simulink model "c00004M_harness"  (R2018a)
settings: Solver=FixedStepAuto  StartTime=0.0  StopTime=300  FixedStep=0.1  RelTol=1e-3
undefined symbols (not defined in the file): A1, hmax, R1, R2, sigbuilder_block, TempThreshold
(part 2 of 14)

== system c00004M_harness/Eval201 ==
  In3 : Inport
  Constant1 : Constant
  Constant2 : Constant
  Data Type Conversion2 : DataTypeConversion
  Memory3 : Memory  InitialCondition=1
  MinMax : MinMax  Inputs=3
  MinMax3 : MinMax  Inputs=2
  ROOut3 : RelationalOperator  Operator===  OutDataTypeStr=boolean  RndMeth=Simplest
  Out1 : Outport
  wires:
  Data Type Conversion2/1 -> MinMax3/1
  Memory3/1 -> MinMax3/2
  ROOut3/1 -> Data Type Conversion2/1
  MinMax3/1 -> Memory3/1, MinMax/3
  In3/1 -> ROOut3/1
  [out3] -> ROOut3/2
  MinMax/1 -> Out1/1
  Constant1/1 -> MinMax/1
  Constant2/1 -> MinMax/2

== system c00004M_harness/Eval202 ==
  In3 : Inport
  Constant1 : Constant
  Constant2 : Constant
  Data Type Conversion2 : DataTypeConversion
  Memory3 : Memory  InitialCondition=1
  MinMax : MinMax  Inputs=3
  MinMax3 : MinMax  Inputs=2
  ROOut3 : RelationalOperator  Operator===  OutDataTypeStr=boolean  RndMeth=Simplest
  Out1 : Outport
  wires:
  Data Type Conversion2/1 -> MinMax3/1
  Memory3/1 -> MinMax3/2
  ROOut3/1 -> Data Type Conversion2/1
  MinMax3/1 -> Memory3/1, MinMax/3
  In3/1 -> ROOut3/1
  [out3] -> ROOut3/2
  MinMax/1 -> Out1/1
  Constant1/1 -> MinMax/1
  Constant2/1 -> MinMax/2

== system c00004M_harness/Eval203 ==
  In3 : Inport
  Constant1 : Constant
  Constant2 : Constant
  Data Type Conversion2 : DataTypeConversion
  Memory3 : Memory  InitialCondition=1
  MinMax : MinMax  Inputs=3
  MinMax3 : MinMax  Inputs=2
  ROOut3 : RelationalOperator  Operator===  OutDataTypeStr=boolean  RndMeth=Simplest
  Out1 : Outport
  wires:
  Data Type Conversion2/1 -> MinMax3/1
  Memory3/1 -> MinMax3/2
  ROOut3/1 -> Data Type Conversion2/1
  MinMax3/1 -> Memory3/1, MinMax/3
  In3/1 -> ROOut3/1
  [out3] -> ROOut3/2
  MinMax/1 -> Out1/1
  Constant1/1 -> MinMax/1
  Constant2/1 -> MinMax/2

== system c00004M_harness/Eval204 ==
  In3 : Inport
  Constant1 : Constant
  Constant2 : Constant
  Data Type Conversion2 : DataTypeConversion
  Memory3 : Memory  InitialCondition=1
  MinMax : MinMax  Inputs=3
  MinMax3 : MinMax  Inputs=2
  ROOut3 : RelationalOperator  Operator===  OutDataTypeStr=boolean  RndMeth=Simplest
  Out1 : Outport
  wires:
  Data Type Conversion2/1 -> MinMax3/1
  Memory3/1 -> MinMax3/2
  ROOut3/1 -> Data Type Conversion2/1
  MinMax3/1 -> Memory3/1, MinMax/3
  In3/1 -> ROOut3/1
  [out3] -> ROOut3/2
  MinMax/1 -> Out1/1
  Constant1/1 -> MinMax/1
  Constant2/1 -> MinMax/2

== system c00004M_harness/Eval205 ==
  In3 : Inport
  Constant1 : Constant
  Constant2 : Constant
  Data Type Conversion2 : DataTypeConversion
  Memory3 : Memory  InitialCondition=1
  MinMax : MinMax  Inputs=3
  MinMax3 : MinMax  Inputs=2
  ROOut3 : RelationalOperator  Operator===  OutDataTypeStr=boolean  RndMeth=Simplest
  Out1 : Outport
  wires:
  Data Type Conversion2/1 -> MinMax3/1
  Memory3/1 -> MinMax3/2
  ROOut3/1 -> Data Type Conversion2/1
  MinMax3/1 -> Memory3/1, MinMax/3
  In3/1 -> ROOut3/1
  [out3] -> ROOut3/2
  MinMax/1 -> Out1/1
  Constant1/1 -> MinMax/1
  Constant2/1 -> MinMax/2

== system c00004M_harness/Eval206 ==
  In3 : Inport
  Constant1 : Constant
  Constant2 : Constant
  Data Type Conversion2 : DataTypeConversion
  Memory3 : Memory  InitialCondition=1
  MinMax : MinMax  Inputs=3
  MinMax3 : MinMax  Inputs=2
  ROOut3 : RelationalOperator  Operator===  OutDataTypeStr=boolean  RndMeth=Simplest
  Out1 : Outport
  wires:
  Data Type Conversion2/1 -> MinMax3/1
  Memory3/1 -> MinMax3/2
  ROOut3/1 -> Data Type Conversion2/1
  MinMax3/1 -> Memory3/1, MinMax/3
  In3/1 -> ROOut3/1
  [out3] -> ROOut3/2
  MinMax/1 -> Out1/1
  Constant1/1 -> MinMax/1
  Constant2/1 -> MinMax/2

== system c00004M_harness/Eval207 ==
  In3 : Inport
  Constant1 : Constant
  Constant2 : Constant
  Data Type Conversion2 : DataTypeConversion
  Memory3 : Memory  InitialCondition=1
  MinMax : MinMax  Inputs=3
  MinMax3 : MinMax  Inputs=2
  ROOut3 : RelationalOperator  Operator===  OutDataTypeStr=boolean  RndMeth=Simplest
  Out1 : Outport
  wires:
  Data Type Conversion2/1 -> MinMax3/1
  Memory3/1 -> MinMax3/2
  ROOut3/1 -> Data Type Conversion2/1
  MinMax3/1 -> Memory3/1, MinMax/3
  In3/1 -> ROOut3/1
  [out3] -> ROOut3/2
  MinMax/1 -> Out1/1
  Constant1/1 -> MinMax/1
  Constant2/1 -> MinMax/2

== system c00004M_harness/Eval208 ==
  In3 : Inport
  Constant1 : Constant
  Constant2 : Constant
  Data Type Conversion2 : DataTypeConversion
  Memory3 : Memory  InitialCondition=1
  MinMax : MinMax  Inputs=3
  MinMax3 : MinMax  Inputs=2
  ROOut3 : RelationalOperator  Operator===  OutDataTypeStr=boolean  RndMeth=Simplest
  Out1 : Outport
  wires:
  Data Type Conversion2/1 -> MinMax3/1
  Memory3/1 -> MinMax3/2
  ROOut3/1 -> Data Type Conversion2/1
  MinMax3/1 -> Memory3/1, MinMax/3
  In3/1 -> ROOut3/1
  [out3] -> ROOut3/2
  MinMax/1 -> Out1/1
  Constant1/1 -> MinMax/1
  Constant2/1 -> MinMax/2

== system c00004M_harness/Eval209 ==
  In3 : Inport
  Constant1 : Constant
  Constant2 : Constant
  Data Type Conversion2 : DataTypeConversion
  Memory3 : Memory  InitialCondition=1
  MinMax : MinMax  Inputs=3
  MinMax3 : MinMax  Inputs=2
  ROOut3 : RelationalOperator  Operator===  OutDataTypeStr=boolean  RndMeth=Simplest
  Out1 : Outport
  wires:
  Data Type Conversion2/1 -> MinMax3/1
  Memory3/1 -> MinMax3/2
  ROOut3/1 -> Data Type Conversion2/1
  MinMax3/1 -> Memory3/1, MinMax/3
  In3/1 -> ROOut3/1
  [out3] -> ROOut3/2
  MinMax/1 -> Out1/1
  Constant1/1 -> MinMax/1
  Constant2/1 -> MinMax/2

== system c00004M_harness/Eval210 ==
  In3 : Inport
  Constant1 : Constant
  Constant2 : Constant
  Data Type Conversion2 : DataTypeConversion
  Memory3 : Memory  InitialCondition=1
  MinMax : MinMax  Inputs=3
  MinMax3 : MinMax  Inputs=2
  ROOut3 : RelationalOperator  Operator===  OutDataTypeStr=boolean  RndMeth=Simplest
  Out1 : Outport
  wires:
  Data Type Conversion2/1 -> MinMax3/1
  Memory3/1 -> MinMax3/2
  ROOut3/1 -> Data Type Conversion2/1
  MinMax3/1 -> Memory3/1, MinMax/3
  In3/1 -> ROOut3/1
  [out3] -> ROOut3/2
  MinMax/1 -> Out1/1
  Constant1/1 -> MinMax/1
  Constant2/1 -> MinMax/2

== system c00004M_harness/Eval211 ==
  In3 : Inport
  Constant1 : Constant
  Constant2 : Constant
  Data Type Conversion2 : DataTypeConversion
  Memory3 : Memory  InitialCondition=1
  MinMax : MinMax  Inputs=3
  MinMax3 : MinMax  Inputs=2
  ROOut3 : RelationalOperator  Operator===  OutDataTypeStr=boolean  RndMeth=Simplest
  Out1 : Outport
  wires:
  Data Type Conversion2/1 -> MinMax3/1
  Memory3/1 -> MinMax3/2
  ROOut3/1 -> Data Type Conversion2/1
  MinMax3/1 -> Memory3/1, MinMax/3
  In3/1 -> ROOut3/1
  [out3] -> ROOut3/2
  MinMax/1 -> Out1/1
  Constant1/1 -> MinMax/1
  Constant2/1 -> MinMax/2

== system c00004M_harness/Eval212 ==
  In3 : Inport
  Constant1 : Constant
  Constant2 : Constant
  Data Type Conversion2 : DataTypeConversion
  Memory3 : Memory  InitialCondition=1
  MinMax : MinMax  Inputs=3
  MinMax3 : MinMax  Inputs=2
  ROOut3 : RelationalOperator  Operator===  OutDataTypeStr=boolean  RndMeth=Simplest
  Out1 : Outport
  wires:
  Data Type Conversion2/1 -> MinMax3/1
  Memory3/1 -> MinMax3/2
  ROOut3/1 -> Data Type Conversion2/1
  MinMax3/1 -> Memory3/1, MinMax/3
  In3/1 -> ROOut3/1
  [out3] -> ROOut3/2
  MinMax/1 -> Out1/1
  Constant1/1 -> MinMax/1
  Constant2/1 -> MinMax/2

== system c00004M_harness/Eval213 ==
  In3 : Inport
  Constant1 : Constant
  Constant2 : Constant
  Data Type Conversion2 : DataTypeConversion
  Memory3 : Memory  InitialCondition=1
  MinMax : MinMax  Inputs=3
  MinMax3 : MinMax  Inputs=2
  ROOut3 : RelationalOperator  Operator===  OutDataTypeStr=boolean  RndMeth=Simplest
  Out1 : Outport
  wires:
  Data Type Conversion2/1 -> MinMax3/1
  Memory3/1 -> MinMax3/2
  ROOut3/1 -> Data Type Conversion2/1
  MinMax3/1 -> Memory3/1, MinMax/3
  In3/1 -> ROOut3/1
  [out3] -> ROOut3/2
  MinMax/1 -> Out1/1
  Constant1/1 -> MinMax/1
  Constant2/1 -> MinMax/2

== system c00004M_harness/Eval214 ==
  In3 : Inport
  Constant1 : Constant
  Constant2 : Constant
  Data Type Conversion2 : DataTypeConversion
  Memory3 : Memory  InitialCondition=1
  MinMax : MinMax  Inputs=3
  MinMax3 : MinMax  Inputs=2
  ROOut3 : RelationalOperator  Operator===  OutDataTypeStr=boolean  RndMeth=Simplest
  Out1 : Outport
  wires:
  Data Type Conversion2/1 -> MinMax3/1
  Memory3/1 -> MinMax3/2
  ROOut3/1 -> Data Type Conversion2/1
  MinMax3/1 -> Memory3/1, MinMax/3
  In3/1 -> ROOut3/1
  [out3] -> ROOut3/2
  MinMax/1 -> Out1/1
  Constant1/1 -> MinMax/1
  Constant2/1 -> MinMax/2

== system c00004M_harness/Eval215 ==
  In3 : Inport
  Constant1 : Constant
  Constant2 : Constant
  Data Type Conversion2 : DataTypeConversion
  Memory3 : Memory  InitialCondition=1
  MinMax : MinMax  Inputs=3
  MinMax3 : MinMax  Inputs=2
  ROOut3 : RelationalOperator  Operator===  OutDataTypeStr=boolean  RndMeth=Simplest
  Out1 : Outport
  wires:
  Data Type Conversion2/1 -> MinMax3/1
  Memory3/1 -> MinMax3/2
  ROOut3/1 -> Data Type Conversion2/1
  MinMax3/1 -> Memory3/1, MinMax/3
  In3/1 -> ROOut3/1
  [out3] -> ROOut3/2
  MinMax/1 -> Out1/1
  Constant1/1 -> MinMax/1
  Constant2/1 -> MinMax/2

== system c00004M_harness/Eval216 ==
  In3 : Inport
  Constant1 : Constant
  Constant2 : Constant
  Data Type Conversion2 : DataTypeConversion
  Memory3 : Memory  InitialCondition=1
  MinMax : MinMax  Inputs=3
  MinMax3 : MinMax  Inputs=2
  ROOut3 : RelationalOperator  Operator===  OutDataTypeStr=boolean  RndMeth=Simplest
  Out1 : Outport
  wires:
  Data Type Conversion2/1 -> MinMax3/1
  Memory3/1 -> MinMax3/2
  ROOut3/1 -> Data Type Conversion2/1
  MinMax3/1 -> Memory3/1, MinMax/3
  In3/1 -> ROOut3/1
  [out3] -> ROOut3/2
  MinMax/1 -> Out1/1
  Constant1/1 -> MinMax/1
  Constant2/1 -> MinMax/2

== system c00004M_harness/Eval217 ==
  In3 : Inport
  Constant1 : Constant
  Constant2 : Constant
  Data Type Conversion2 : DataTypeConversion
  Memory3 : Memory  InitialCondition=1
  MinMax : MinMax  Inputs=3
  MinMax3 : MinMax  Inputs=2
  ROOut3 : RelationalOperator  Operator===  OutDataTypeStr=boolean  RndMeth=Simplest
  Out1 : Outport
  wires:
  Data Type Conversion2/1 -> MinMax3/1
  Memory3/1 -> MinMax3/2
  ROOut3/1 -> Data Type Conversion2/1
  MinMax3/1 -> Memory3/1, MinMax/3
  In3/1 -> ROOut3/1
  [out3] -> ROOut3/2
  MinMax/1 -> Out1/1
  Constant1/1 -> MinMax/1
  Constant2/1 -> MinMax/2

== system c00004M_harness/Eval218 ==
  In3 : Inport
  Constant1 : Constant
  Constant2 : Constant
  Data Type Conversion2 : DataTypeConversion
  Memory3 : Memory  InitialCondition=1
  MinMax : MinMax  Inputs=3
  MinMax3 : MinMax  Inputs=2
  ROOut3 : RelationalOperator  Operator===  OutDataTypeStr=boolean  RndMeth=Simplest
  Out1 : Outport
  wires:
  Data Type Conversion2/1 -> MinMax3/1
  Memory3/1 -> MinMax3/2
  ROOut3/1 -> Data Type Conversion2/1
  MinMax3/1 -> Memory3/1, MinMax/3
  In3/1 -> ROOut3/1
  [out3] -> ROOut3/2
  MinMax/1 -> Out1/1
  Constant1/1 -> MinMax/1
  Constant2/1 -> MinMax/2

== system c00004M_harness/Eval219 ==
  In3 : Inport
  Constant1 : Constant
  Constant2 : Constant
  Data Type Conversion2 : DataTypeConversion
  Memory3 : Memory  InitialCondition=1
  MinMax : MinMax  Inputs=3
  MinMax3 : MinMax  Inputs=2
  ROOut3 : RelationalOperator  Operator===  OutDataTypeStr=boolean  RndMeth=Simplest
  Out1 : Outport
  wires:
  Data Type Conversion2/1 -> MinMax3/1
  Memory3/1 -> MinMax3/2
  ROOut3/1 -> Data Type Conversion2/1
  MinMax3/1 -> Memory3/1, MinMax/3
  In3/1 -> ROOut3/1
  [out3] -> ROOut3/2
  MinMax/1 -> Out1/1
  Constant1/1 -> MinMax/1
  Constant2/1 -> MinMax/2

== system c00004M_harness/Eval220 ==
  In3 : Inport
  Constant1 : Constant
  Constant2 : Constant
  Data Type Conversion2 : DataTypeConversion
  Memory3 : Memory  InitialCondition=1
  MinMax : MinMax  Inputs=3
  MinMax3 : MinMax  Inputs=2
  ROOut3 : RelationalOperator  Operator===  OutDataTypeStr=boolean  RndMeth=Simplest
  Out1 : Outport
  wires:
  Data Type Conversion2/1 -> MinMax3/1
  Memory3/1 -> MinMax3/2
  ROOut3/1 -> Data Type Conversion2/1
  MinMax3/1 -> Memory3/1, MinMax/3
  In3/1 -> ROOut3/1
  [out3] -> ROOut3/2
  MinMax/1 -> Out1/1
  Constant1/1 -> MinMax/1
  Constant2/1 -> MinMax/2

== system c00004M_harness/Eval221 ==
  In3 : Inport
  Constant1 : Constant
  Constant2 : Constant
  Data Type Conversion2 : DataTypeConversion
  Memory3 : Memory  InitialCondition=1
  MinMax : MinMax  Inputs=3
  MinMax3 : MinMax  Inputs=2
  ROOut3 : RelationalOperator  Operator===  OutDataTypeStr=boolean  RndMeth=Simplest
  Out1 : Outport
  wires:
  Data Type Conversion2/1 -> MinMax3/1
  Memory3/1 -> MinMax3/2
  ROOut3/1 -> Data Type Conversion2/1
  MinMax3/1 -> Memory3/1, MinMax/3
  In3/1 -> ROOut3/1
  [out3] -> ROOut3/2
  MinMax/1 -> Out1/1
  Constant1/1 -> MinMax/1
  Constant2/1 -> MinMax/2

== system c00004M_harness/Eval222 ==
  In3 : Inport
  Constant1 : Constant
  Constant2 : Constant
  Data Type Conversion2 : DataTypeConversion
  Memory3 : Memory  InitialCondition=1
  MinMax : MinMax  Inputs=3
  MinMax3 : MinMax  Inputs=2
  ROOut3 : RelationalOperator  Operator===  OutDataTypeStr=boolean  RndMeth=Simplest
  Out1 : Outport
  wires:
  Data Type Conversion2/1 -> MinMax3/1
  Memory3/1 -> MinMax3/2
  ROOut3/1 -> Data Type Conversion2/1
  MinMax3/1 -> Memory3/1, MinMax/3
  In3/1 -> ROOut3/1
  [out3] -> ROOut3/2
  MinMax/1 -> Out1/1
  Constant1/1 -> MinMax/1
  Constant2/1 -> MinMax/2

== system c00004M_harness/Eval223 ==
  In3 : Inport
  Constant1 : Constant
  Constant2 : Constant
  Data Type Conversion2 : DataTypeConversion
  Memory3 : Memory  InitialCondition=1
  MinMax : MinMax  Inputs=3
  MinMax3 : MinMax  Inputs=2
  ROOut3 : RelationalOperator  Operator===  OutDataTypeStr=boolean  RndMeth=Simplest
  Out1 : Outport
  wires:
  Data Type Conversion2/1 -> MinMax3/1
  Memory3/1 -> MinMax3/2
  ROOut3/1 -> Data Type Conversion2/1
  MinMax3/1 -> Memory3/1, MinMax/3
  In3/1 -> ROOut3/1
  [out3] -> ROOut3/2
  MinMax/1 -> Out1/1
  Constant1/1 -> MinMax/1
  Constant2/1 -> MinMax/2

== system c00004M_harness/Eval224 ==
  In3 : Inport
  Constant1 : Constant
  Constant2 : Constant
  Data Type Conversion2 : DataTypeConversion
  Memory3 : Memory  InitialCondition=1
  MinMax : MinMax  Inputs=3
  MinMax3 : MinMax  Inputs=2
  ROOut3 : RelationalOperator  Operator===  OutDataTypeStr=boolean  RndMeth=Simplest
  Out1 : Outport
  wires:
  Data Type Conversion2/1 -> MinMax3/1
  Memory3/1 -> MinMax3/2
  ROOut3/1 -> Data Type Conversion2/1
  MinMax3/1 -> Memory3/1, MinMax/3
  In3/1 -> ROOut3/1
  [out3] -> ROOut3/2
  MinMax/1 -> Out1/1
  Constant1/1 -> MinMax/1
  Constant2/1 -> MinMax/2

== system c00004M_harness/Eval232 ==
  In3 : Inport
  Constant1 : Constant
  Constant2 : Constant
  Data Type Conversion2 : DataTypeConversion
  Memory3 : Memory  InitialCondition=1
  MinMax : MinMax  Inputs=3
  MinMax3 : MinMax  Inputs=2
  ROOut3 : RelationalOperator  Operator===  OutDataTypeStr=boolean  RndMeth=Simplest
  Out1 : Outport
  wires:
  Data Type Conversion2/1 -> MinMax3/1
  Memory3/1 -> MinMax3/2
  ROOut3/1 -> Data Type Conversion2/1
  MinMax3/1 -> Memory3/1, MinMax/3
  In3/1 -> ROOut3/1
  [out3] -> ROOut3/2
  MinMax/1 -> Out1/1
  Constant1/1 -> MinMax/1
  Constant2/1 -> MinMax/2

== system c00004M_harness/Eval233 ==
  In3 : Inport
  Constant1 : Constant
  Constant2 : Constant
  Data Type Conversion2 : DataTypeConversion
  Memory3 : Memory  InitialCondition=1
  MinMax : MinMax  Inputs=3
  MinMax3 : MinMax  Inputs=2
  ROOut3 : RelationalOperator  Operator===  OutDataTypeStr=boolean  RndMeth=Simplest
  Out1 : Outport
  wires:
  Data Type Conversion2/1 -> MinMax3/1
  Memory3/1 -> MinMax3/2
  ROOut3/1 -> Data Type Conversion2/1
  MinMax3/1 -> Memory3/1, MinMax/3
  In3/1 -> ROOut3/1
  [out3] -> ROOut3/2
  MinMax/1 -> Out1/1
  Constant1/1 -> MinMax/1
  Constant2/1 -> MinMax/2

== system c00004M_harness/Eval234 ==
  In3 : Inport
  Constant1 : Constant
  Constant2 : Constant
  Data Type Conversion2 : DataTypeConversion
  Memory3 : Memory  InitialCondition=1
  MinMax : MinMax  Inputs=3
  MinMax3 : MinMax  Inputs=2
  ROOut3 : RelationalOperator  Operator===  OutDataTypeStr=boolean  RndMeth=Simplest
  Out1 : Outport
  wires:
  Data Type Conversion2/1 -> MinMax3/1
  Memory3/1 -> MinMax3/2
  ROOut3/1 -> Data Type Conversion2/1
  MinMax3/1 -> Memory3/1, MinMax/3
  In3/1 -> ROOut3/1
  [out3] -> ROOut3/2
  MinMax/1 -> Out1/1
  Constant1/1 -> MinMax/1
  Constant2/1 -> MinMax/2

== system c00004M_harness/Eval235 ==
  In3 : Inport
  Constant1 : Constant
  Constant2 : Constant
  Data Type Conversion2 : DataTypeConversion
  Memory3 : Memory  InitialCondition=1
  MinMax : MinMax  Inputs=3
  MinMax3 : MinMax  Inputs=2
  ROOut3 : RelationalOperator  Operator===  OutDataTypeStr=boolean  RndMeth=Simplest
  Out1 : Outport
  wires:
  Data Type Conversion2/1 -> MinMax3/1
  Memory3/1 -> MinMax3/2
  ROOut3/1 -> Data Type Conversion2/1
  MinMax3/1 -> Memory3/1, MinMax/3
  In3/1 -> ROOut3/1
  [out3] -> ROOut3/2
  MinMax/1 -> Out1/1
  Constant1/1 -> MinMax/1
  Constant2/1 -> MinMax/2

== system c00004M_harness/Eval236 ==
  In3 : Inport
  Constant1 : Constant
  Constant2 : Constant
  Data Type Conversion2 : DataTypeConversion
  Memory3 : Memory  InitialCondition=1
  MinMax : MinMax  Inputs=3
  MinMax3 : MinMax  Inputs=2
  ROOut3 : RelationalOperator  Operator===  OutDataTypeStr=boolean  RndMeth=Simplest
  Out1 : Outport
  wires:
  Data Type Conversion2/1 -> MinMax3/1
  Memory3/1 -> MinMax3/2
  ROOut3/1 -> Data Type Conversion2/1
  MinMax3/1 -> Memory3/1, MinMax/3
  In3/1 -> ROOut3/1
  [out3] -> ROOut3/2
  MinMax/1 -> Out1/1
  Constant1/1 -> MinMax/1
  Constant2/1 -> MinMax/2

== system c00004M_harness/Eval237 ==
  In3 : Inport
  Constant1 : Constant
  Constant2 : Constant
  Data Type Conversion2 : DataTypeConversion
  Memory3 : Memory  InitialCondition=1
  MinMax : MinMax  Inputs=3
  MinMax3 : MinMax  Inputs=2
  ROOut3 : RelationalOperator  Operator===  OutDataTypeStr=boolean  RndMeth=Simplest
  Out1 : Outport
  wires:
  Data Type Conversion2/1 -> MinMax3/1
  Memory3/1 -> MinMax3/2
  ROOut3/1 -> Data Type Conversion2/1
  MinMax3/1 -> Memory3/1, MinMax/3
  In3/1 -> ROOut3/1
  [out3] -> ROOut3/2
  MinMax/1 -> Out1/1
  Constant1/1 -> MinMax/1
  Constant2/1 -> MinMax/2

== system c00004M_harness/Eval238 ==
  In3 : Inport
  Constant1 : Constant
  Constant2 : Constant
  Data Type Conversion2 : DataTypeConversion
  Memory3 : Memory  InitialCondition=1
  MinMax : MinMax  Inputs=3
  MinMax3 : MinMax  Inputs=2
  ROOut3 : RelationalOperator  Operator===  OutDataTypeStr=boolean  RndMeth=Simplest
  Out1 : Outport
  wires:
  Data Type Conversion2/1 -> MinMax3/1
  Memory3/1 -> MinMax3/2
  ROOut3/1 -> Data Type Conversion2/1
  MinMax3/1 -> Memory3/1, MinMax/3
  In3/1 -> ROOut3/1
  [out3] -> ROOut3/2
  MinMax/1 -> Out1/1
  Constant1/1 -> MinMax/1
  Constant2/1 -> MinMax/2

== system c00004M_harness/Eval239 ==
  In3 : Inport
  Constant1 : Constant
  Constant2 : Constant
  Data Type Conversion2 : DataTypeConversion
  Memory3 : Memory  InitialCondition=1
  MinMax : MinMax  Inputs=3
  MinMax3 : MinMax  Inputs=2
  ROOut3 : RelationalOperator  Operator===  OutDataTypeStr=boolean  RndMeth=Simplest
  Out1 : Outport
  wires:
  Data Type Conversion2/1 -> MinMax3/1
  Memory3/1 -> MinMax3/2
  ROOut3/1 -> Data Type Conversion2/1
  MinMax3/1 -> Memory3/1, MinMax/3
  In3/1 -> ROOut3/1
  [out3] -> ROOut3/2
  MinMax/1 -> Out1/1
  Constant1/1 -> MinMax/1
  Constant2/1 -> MinMax/2

== system c00004M_harness/Eval240 ==
  In3 : Inport
  Constant1 : Constant
  Constant2 : Constant
  Data Type Conversion2 : DataTypeConversion
  Memory3 : Memory  InitialCondition=1
  MinMax : MinMax  Inputs=3
  MinMax3 : MinMax  Inputs=2
  ROOut3 : RelationalOperator  Operator===  OutDataTypeStr=boolean  RndMeth=Simplest
  Out1 : Outport
  wires:
  Data Type Conversion2/1 -> MinMax3/1
  Memory3/1 -> MinMax3/2
  ROOut3/1 -> Data Type Conversion2/1
  MinMax3/1 -> Memory3/1, MinMax/3
  In3/1 -> ROOut3/1
  [out3] -> ROOut3/2
  MinMax/1 -> Out1/1
  Constant1/1 -> MinMax/1
  Constant2/1 -> MinMax/2

== system c00004M_harness/Eval241 ==
  In3 : Inport
  Constant1 : Constant
  Constant2 : Constant
  Data Type Conversion2 : DataTypeConversion
  Memory3 : Memory  InitialCondition=1
  MinMax : MinMax  Inputs=3
  MinMax3 : MinMax  Inputs=2
  ROOut3 : RelationalOperator  Operator===  OutDataTypeStr=boolean  RndMeth=Simplest
  Out1 : Outport
  wires:
  Data Type Conversion2/1 -> MinMax3/1
  Memory3/1 -> MinMax3/2
  ROOut3/1 -> Data Type Conversion2/1
  MinMax3/1 -> Memory3/1, MinMax/3
  In3/1 -> ROOut3/1
  [out3] -> ROOut3/2
  MinMax/1 -> Out1/1
  Constant1/1 -> MinMax/1
  Constant2/1 -> MinMax/2

== system c00004M_harness/Eval242 ==
  In3 : Inport
  Constant1 : Constant
  Constant2 : Constant
  Data Type Conversion2 : DataTypeConversion
  Memory3 : Memory  InitialCondition=1
  MinMax : MinMax  Inputs=3
  MinMax3 : MinMax  Inputs=2
  ROOut3 : RelationalOperator  Operator===  OutDataTypeStr=boolean  RndMeth=Simplest
  Out1 : Outport
  wires:
  Data Type Conversion2/1 -> MinMax3/1
  Memory3/1 -> MinMax3/2
  ROOut3/1 -> Data Type Conversion2/1
  MinMax3/1 -> Memory3/1, MinMax/3
  In3/1 -> ROOut3/1
  [out3] -> ROOut3/2
  MinMax/1 -> Out1/1
  Constant1/1 -> MinMax/1
  Constant2/1 -> MinMax/2

== system c00004M_harness/Eval243 ==
  In3 : Inport
  Constant1 : Constant
  Constant2 : Constant
  Data Type Conversion2 : DataTypeConversion
  Memory3 : Memory  InitialCondition=1
  MinMax : MinMax  Inputs=3
  MinMax3 : MinMax  Inputs=2
  ROOut3 : RelationalOperator  Operator===  OutDataTypeStr=boolean  RndMeth=Simplest
  Out1 : Outport
  wires:
  Data Type Conversion2/1 -> MinMax3/1
  Memory3/1 -> MinMax3/2
  ROOut3/1 -> Data Type Conversion2/1
  MinMax3/1 -> Memory3/1, MinMax/3
  In3/1 -> ROOut3/1
  [out3] -> ROOut3/2
  MinMax/1 -> Out1/1
  Constant1/1 -> MinMax/1
  Constant2/1 -> MinMax/2

== system c00004M_harness/Eval244 ==
  In3 : Inport
  Constant1 : Constant
  Constant2 : Constant
  Data Type Conversion2 : DataTypeConversion
  Memory3 : Memory  InitialCondition=1
  MinMax : MinMax  Inputs=3
  MinMax3 : MinMax  Inputs=2
  ROOut3 : RelationalOperator  Operator===  OutDataTypeStr=boolean  RndMeth=Simplest
  Out1 : Outport
  wires:
  Data Type Conversion2/1 -> MinMax3/1
  Memory3/1 -> MinMax3/2
  ROOut3/1 -> Data Type Conversion2/1
  MinMax3/1 -> Memory3/1, MinMax/3
  In3/1 -> ROOut3/1
  [out3] -> ROOut3/2
  MinMax/1 -> Out1/1
  Constant1/1 -> MinMax/1
  Constant2/1 -> MinMax/2

== system c00004M_harness/Eval245 ==
  In3 : Inport
  Constant1 : Constant
  Constant2 : Constant
  Data Type Conversion2 : DataTypeConversion
  Memory3 : Memory  InitialCondition=1
  MinMax : MinMax  Inputs=3
  MinMax3 : MinMax  Inputs=2
  ROOut3 : RelationalOperator  Operator===  OutDataTypeStr=boolean  RndMeth=Simplest
  Out1 : Outport
  wires:
  Data Type Conversion2/1 -> MinMax3/1
  Memory3/1 -> MinMax3/2
  ROOut3/1 -> Data Type Conversion2/1
  MinMax3/1 -> Memory3/1, MinMax/3
  In3/1 -> ROOut3/1
  [out3] -> ROOut3/2
  MinMax/1 -> Out1/1
  Constant1/1 -> MinMax/1
  Constant2/1 -> MinMax/2

== system c00004M_harness/Inputs ==
  Demux : Demux  Tag=STV Demux  Outputs=6
  FromWs : FromWorkspace  Tag=STV FromWs  VariableName=tuvar  SampleTime=0
  CT3 : Outport  Tag=STV Outport
  F3 : Outport  Tag=STV Outport  Port=2
  E3 : Outport  Tag=STV Outport  Port=3
  MR3 : Outport  Tag=STV Outport  Port=4
  T3 : Outport  Tag=STV Outport  Port=5
  EB3 : Outport  Tag=STV Outport  Port=6
  wires:
  Demux/6 -> EB3/1
  Demux/5 -> T3/1
  Demux/4 -> MR3/1
  Demux/3 -> E3/1
  Demux/2 -> F3/1
  Demux/1 -> CT3/1
  FromWs/1 -> Demux/1

== system c00004M_harness/M165 ==
  note: VALUES
      | ---------------------------------
      | ControlType = 1 | 2 | 3
      | FillTank = 0 | 1
      | EmptyTank = 0 | 1
      | ManualReference between 0 and 1
      | Tempreature between 0 and 100
      | EmergencyButton = 0 | 1
      | LiquidLevel between 0 and 1 (hmax)
  note: Inputs For Tank2
  note: NAMES
      | --------------------------------------------
      | CT1 = ControlType Tank 1
      | F1 = Fill Tank 1
      | E1 = Empty Tank 1
      | MR1 = Manual Reference Tank1
      | T1 = Temperature Tank 1
      | EB1 = Emergency Button Tank 1
      | LL1 = Liquid Level 1
  note: Inputs For Tank3
  note: Inputs For Tank1
  CT3 : Inport
  F3 : Inport  Port=2
  E3 : Inport  Port=3
  MR3 : Inport  Port=4
  T3 : Inport  Port=5
  EB3 : Inport  Port=6
  Tank3 : Subsystem
  LL3 : Outport
  wires:
  Tank3/1(LL3) -> LL3/1
  MR3/1 -> Tank3/4(MR3)
  E3/1 -> Tank3/3(E3)
  CT3/1 -> Tank3/1(CT3)
  F3/1 -> Tank3/2(F3)
  EB3/1 -> Tank3/6(EB3)
  T3/1 -> Tank3/5(T3)

== system c00004M_harness/M166 ==
  note: VALUES
      | ---------------------------------
      | ControlType = 1 | 2 | 3
      | FillTank = 0 | 1
      | EmptyTank = 0 | 1
      | ManualReference between 0 and 1
      | Tempreature between 0 and 100
      | EmergencyButton = 0 | 1
      | LiquidLevel between 0 and 1 (hmax)
  note: Inputs For Tank2
  note: NAMES
      | --------------------------------------------
      | CT1 = ControlType Tank 1
      | F1 = Fill Tank 1
      | E1 = Empty Tank 1
      | MR1 = Manual Reference Tank1
      | T1 = Temperature Tank 1
      | EB1 = Emergency Button Tank 1
      | LL1 = Liquid Level 1
  note: Inputs For Tank3
  note: Inputs For Tank1
  CT3 : Inport
  F3 : Inport  Port=2
  E3 : Inport  Port=3
  MR3 : Inport  Port=4
  T3 : Inport  Port=5
  EB3 : Inport  Port=6
  Tank3 : Subsystem
  LL3 : Outport
  wires:
  Tank3/1(LL3) -> LL3/1
  MR3/1 -> Tank3/4(MR3)
  E3/1 -> Tank3/3(E3)
  CT3/1 -> Tank3/1(CT3)
  F3/1 -> Tank3/2(F3)
  EB3/1 -> Tank3/6(EB3)
  T3/1 -> Tank3/5(T3)

== system c00004M_harness/M167 ==
  note: VALUES
      | ---------------------------------
      | ControlType = 1 | 2 | 3
      | FillTank = 0 | 1
      | EmptyTank = 0 | 1
      | ManualReference between 0 and 1
      | Tempreature between 0 and 100
      | EmergencyButton = 0 | 1
      | LiquidLevel between 0 and 1 (hmax)
  note: Inputs For Tank2
  note: NAMES
      | --------------------------------------------
      | CT1 = ControlType Tank 1
      | F1 = Fill Tank 1
      | E1 = Empty Tank 1
      | MR1 = Manual Reference Tank1
      | T1 = Temperature Tank 1
      | EB1 = Emergency Button Tank 1
      | LL1 = Liquid Level 1
  note: Inputs For Tank3
  note: Inputs For Tank1
  CT3 : Inport
  F3 : Inport  Port=2
  E3 : Inport  Port=3
  MR3 : Inport  Port=4
  T3 : Inport  Port=5
  EB3 : Inport  Port=6
  Tank3 : Subsystem
  LL3 : Outport
  wires:
  Tank3/1(LL3) -> LL3/1
  MR3/1 -> Tank3/4(MR3)
  E3/1 -> Tank3/3(E3)
  CT3/1 -> Tank3/1(CT3)
  F3/1 -> Tank3/2(F3)
  EB3/1 -> Tank3/6(EB3)
  T3/1 -> Tank3/5(T3)

== system c00004M_harness/M168 ==
  note: VALUES
      | ---------------------------------
      | ControlType = 1 | 2 | 3
      | FillTank = 0 | 1
      | EmptyTank = 0 | 1
      | ManualReference between 0 and 1
      | Tempreature between 0 and 100
      | EmergencyButton = 0 | 1
      | LiquidLevel between 0 and 1 (hmax)
  note: Inputs For Tank2
  note: NAMES
      | --------------------------------------------
      | CT1 = ControlType Tank 1
      | F1 = Fill Tank 1
      | E1 = Empty Tank 1
      | MR1 = Manual Reference Tank1
      | T1 = Temperature Tank 1
      | EB1 = Emergency Button Tank 1
      | LL1 = Liquid Level 1
  note: Inputs For Tank3
  note: Inputs For Tank1
  CT3 : Inport
  F3 : Inport  Port=2
  E3 : Inport  Port=3
  MR3 : Inport  Port=4
  T3 : Inport  Port=5
  EB3 : Inport  Port=6
  Tank3 : Subsystem
  LL3 : Outport
  wires:
  Tank3/1(LL3) -> LL3/1
  MR3/1 -> Tank3/4(MR3)
  E3/1 -> Tank3/3(E3)
  CT3/1 -> Tank3/1(CT3)
  F3/1 -> Tank3/2(F3)
  EB3/1 -> Tank3/6(EB3)
  T3/1 -> Tank3/5(T3)

== system c00004M_harness/M169 ==
  note: VALUES
      | ---------------------------------
      | ControlType = 1 | 2 | 3
      | FillTank = 0 | 1
      | EmptyTank = 0 | 1
      | ManualReference between 0 and 1
      | Tempreature between 0 and 100
      | EmergencyButton = 0 | 1
      | LiquidLevel between 0 and 1 (hmax)
  note: Inputs For Tank2
  note: NAMES
      | --------------------------------------------
      | CT1 = ControlType Tank 1
      | F1 = Fill Tank 1
      | E1 = Empty Tank 1
      | MR1 = Manual Reference Tank1
      | T1 = Temperature Tank 1
      | EB1 = Emergency Button Tank 1
      | LL1 = Liquid Level 1
  note: Inputs For Tank3
  note: Inputs For Tank1
  CT3 : Inport
  F3 : Inport  Port=2
  E3 : Inport  Port=3
  MR3 : Inport  Port=4
  T3 : Inport  Port=5
  EB3 : Inport  Port=6
  Tank3 : Subsystem
  LL3 : Outport
  wires:
  Tank3/1(LL3) -> LL3/1
  MR3/1 -> Tank3/4(MR3)
  E3/1 -> Tank3/3(E3)
  CT3/1 -> Tank3/1(CT3)
  F3/1 -> Tank3/2(F3)
  EB3/1 -> Tank3/6(EB3)
  T3/1 -> Tank3/5(T3)

== system c00004M_harness/M170 ==
  note: VALUES
      | ---------------------------------
      | ControlType = 1 | 2 | 3
      | FillTank = 0 | 1
      | EmptyTank = 0 | 1
      | ManualReference between 0 and 1
      | Tempreature between 0 and 100
      | EmergencyButton = 0 | 1
      | LiquidLevel between 0 and 1 (hmax)
  note: Inputs For Tank2
  note: NAMES
      | --------------------------------------------
      | CT1 = ControlType Tank 1
      | F1 = Fill Tank 1
      | E1 = Empty Tank 1
      | MR1 = Manual Reference Tank1
      | T1 = Temperature Tank 1
      | EB1 = Emergency Button Tank 1
      | LL1 = Liquid Level 1
  note: Inputs For Tank3
  note: Inputs For Tank1
  CT3 : Inport
  F3 : Inport  Port=2
  E3 : Inport  Port=3
  MR3 : Inport  Port=4
  T3 : Inport  Port=5
  EB3 : Inport  Port=6
  Tank3 : Subsystem
  LL3 : Outport
  wires:
  Tank3/1(LL3) -> LL3/1
  MR3/1 -> Tank3/4(MR3)
  E3/1 -> Tank3/3(E3)
  CT3/1 -> Tank3/1(CT3)
  F3/1 -> Tank3/2(F3)
  EB3/1 -> Tank3/6(EB3)
  T3/1 -> Tank3/5(T3)

== system c00004M_harness/M171 ==
  note: VALUES
      | ---------------------------------
      | ControlType = 1 | 2 | 3
      | FillTank = 0 | 1
      | EmptyTank = 0 | 1
      | ManualReference between 0 and 1
      | Tempreature between 0 and 100
      | EmergencyButton = 0 | 1
      | LiquidLevel between 0 and 1 (hmax)
  note: Inputs For Tank2
  note: NAMES
      | --------------------------------------------
      | CT1 = ControlType Tank 1
      | F1 = Fill Tank 1
      | E1 = Empty Tank 1
      | MR1 = Manual Reference Tank1
      | T1 = Temperature Tank 1
      | EB1 = Emergency Button Tank 1
      | LL1 = Liquid Level 1
  note: Inputs For Tank3
  note: Inputs For Tank1
  CT3 : Inport
  F3 : Inport  Port=2
  E3 : Inport  Port=3
  MR3 : Inport  Port=4
  T3 : Inport  Port=5
  EB3 : Inport  Port=6
  Tank3 : Subsystem
  LL3 : Outport
  wires:
  Tank3/1(LL3) -> LL3/1
  MR3/1 -> Tank3/4(MR3)
  E3/1 -> Tank3/3(E3)
  CT3/1 -> Tank3/1(CT3)
  F3/1 -> Tank3/2(F3)
  EB3/1 -> Tank3/6(EB3)
  T3/1 -> Tank3/5(T3)

== system c00004M_harness/M172 ==
  note: VALUES
      | ---------------------------------
      | ControlType = 1 | 2 | 3
      | FillTank = 0 | 1
      | EmptyTank = 0 | 1
      | ManualReference between 0 and 1
      | Tempreature between 0 and 100
      | EmergencyButton = 0 | 1
      | LiquidLevel between 0 and 1 (hmax)
  note: Inputs For Tank2
  note: NAMES
      | --------------------------------------------
      | CT1 = ControlType Tank 1
      | F1 = Fill Tank 1
      | E1 = Empty Tank 1
      | MR1 = Manual Reference Tank1
      | T1 = Temperature Tank 1
      | EB1 = Emergency Button Tank 1
      | LL1 = Liquid Level 1
  note: Inputs For Tank3
  note: Inputs For Tank1
  CT3 : Inport
  F3 : Inport  Port=2
  E3 : Inport  Port=3
  MR3 : Inport  Port=4
  T3 : Inport  Port=5
  EB3 : Inport  Port=6
  Tank3 : Subsystem
  LL3 : Outport
  wires:
  Tank3/1(LL3) -> LL3/1
  MR3/1 -> Tank3/4(MR3)
  E3/1 -> Tank3/3(E3)
  CT3/1 -> Tank3/1(CT3)
  F3/1 -> Tank3/2(F3)
  EB3/1 -> Tank3/6(EB3)
  T3/1 -> Tank3/5(T3)

== system c00004M_harness/M173 ==
  note: VALUES
      | ---------------------------------
      | ControlType = 1 | 2 | 3
      | FillTank = 0 | 1
      | EmptyTank = 0 | 1
      | ManualReference between 0 and 1
      | Tempreature between 0 and 100
      | EmergencyButton = 0 | 1
      | LiquidLevel between 0 and 1 (hmax)
  note: Inputs For Tank2
  note: NAMES
      | --------------------------------------------
      | CT1 = ControlType Tank 1
      | F1 = Fill Tank 1
      | E1 = Empty Tank 1
      | MR1 = Manual Reference Tank1
      | T1 = Temperature Tank 1
      | EB1 = Emergency Button Tank 1
      | LL1 = Liquid Level 1
  note: Inputs For Tank3
  note: Inputs For Tank1
  CT3 : Inport
  F3 : Inport  Port=2
  E3 : Inport  Port=3
  MR3 : Inport  Port=4
  T3 : Inport  Port=5
  EB3 : Inport  Port=6
  Tank3 : Subsystem
  LL3 : Outport
  wires:
  Tank3/1(LL3) -> LL3/1
  MR3/1 -> Tank3/4(MR3)
  E3/1 -> Tank3/3(E3)
  CT3/1 -> Tank3/1(CT3)
  F3/1 -> Tank3/2(F3)
  EB3/1 -> Tank3/6(EB3)
  T3/1 -> Tank3/5(T3)

== system c00004M_harness/M174 ==
  note: VALUES
      | ---------------------------------
      | ControlType = 1 | 2 | 3
      | FillTank = 0 | 1
      | EmptyTank = 0 | 1
      | ManualReference between 0 and 1
      | Tempreature between 0 and 100
      | EmergencyButton = 0 | 1
      | LiquidLevel between 0 and 1 (hmax)
  note: Inputs For Tank2
  note: NAMES
      | --------------------------------------------
      | CT1 = ControlType Tank 1
      | F1 = Fill Tank 1
      | E1 = Empty Tank 1
      | MR1 = Manual Reference Tank1
      | T1 = Temperature Tank 1
      | EB1 = Emergency Button Tank 1
      | LL1 = Liquid Level 1
  note: Inputs For Tank3
  note: Inputs For Tank1
  CT3 : Inport
  F3 : Inport  Port=2
  E3 : Inport  Port=3
  MR3 : Inport  Port=4
  T3 : Inport  Port=5
  EB3 : Inport  Port=6
  Tank3 : Subsystem
  LL3 : Outport
  wires:
  Tank3/1(LL3) -> LL3/1
  MR3/1 -> Tank3/4(MR3)
  E3/1 -> Tank3/3(E3)
  CT3/1 -> Tank3/1(CT3)
  F3/1 -> Tank3/2(F3)
  EB3/1 -> Tank3/6(EB3)
  T3/1 -> Tank3/5(T3)

== system c00004M_harness/M175 ==
  note: VALUES
      | ---------------------------------
      | ControlType = 1 | 2 | 3
      | FillTank = 0 | 1
      | EmptyTank = 0 | 1
      | ManualReference between 0 and 1
      | Tempreature between 0 and 100
      | EmergencyButton = 0 | 1
      | LiquidLevel between 0 and 1 (hmax)
  note: Inputs For Tank2
  note: NAMES
      | --------------------------------------------
      | CT1 = ControlType Tank 1
      | F1 = Fill Tank 1
      | E1 = Empty Tank 1
      | MR1 = Manual Reference Tank1
      | T1 = Temperature Tank 1
      | EB1 = Emergency Button Tank 1
      | LL1 = Liquid Level 1
  note: Inputs For Tank3
  note: Inputs For Tank1
  CT3 : Inport
  F3 : Inport  Port=2
  E3 : Inport  Port=3
  MR3 : Inport  Port=4
  T3 : Inport  Port=5
  EB3 : Inport  Port=6
  Tank3 : Subsystem
  LL3 : Outport
  wires:
  Tank3/1(LL3) -> LL3/1
  MR3/1 -> Tank3/4(MR3)
  E3/1 -> Tank3/3(E3)
  CT3/1 -> Tank3/1(CT3)
  F3/1 -> Tank3/2(F3)
  EB3/1 -> Tank3/6(EB3)
  T3/1 -> Tank3/5(T3)

== system c00004M_harness/M176 ==
  note: VALUES
      | ---------------------------------
      | ControlType = 1 | 2 | 3
      | FillTank = 0 | 1
      | EmptyTank = 0 | 1
      | ManualReference between 0 and 1
      | Tempreature between 0 and 100
      | EmergencyButton = 0 | 1
      | LiquidLevel between 0 and 1 (hmax)
  note: Inputs For Tank2
  note: NAMES
      | --------------------------------------------
      | CT1 = ControlType Tank 1
      | F1 = Fill Tank 1
      | E1 = Empty Tank 1
      | MR1 = Manual Reference Tank1
      | T1 = Temperature Tank 1
      | EB1 = Emergency Button Tank 1
      | LL1 = Liquid Level 1
  note: Inputs For Tank3
  note: Inputs For Tank1
  CT3 : Inport
  F3 : Inport  Port=2
  E3 : Inport  Port=3
  MR3 : Inport  Port=4
  T3 : Inport  Port=5
  EB3 : Inport  Port=6
  Tank3 : Subsystem
  LL3 : Outport
  wires:
  Tank3/1(LL3) -> LL3/1
  MR3/1 -> Tank3/4(MR3)
  E3/1 -> Tank3/3(E3)
  CT3/1 -> Tank3/1(CT3)
  F3/1 -> Tank3/2(F3)
  EB3/1 -> Tank3/6(EB3)
  T3/1 -> Tank3/5(T3)

== system c00004M_harness/M177 ==
  note: VALUES
      | ---------------------------------
      | ControlType = 1 | 2 | 3
      | FillTank = 0 | 1
      | EmptyTank = 0 | 1
      | ManualReference between 0 and 1
      | Tempreature between 0 and 100
      | EmergencyButton = 0 | 1
      | LiquidLevel between 0 and 1 (hmax)
  note: Inputs For Tank2
  note: NAMES
      | --------------------------------------------
      | CT1 = ControlType Tank 1
      | F1 = Fill Tank 1
      | E1 = Empty Tank 1
      | MR1 = Manual Reference Tank1
      | T1 = Temperature Tank 1
      | EB1 = Emergency Button Tank 1
      | LL1 = Liquid Level 1
  note: Inputs For Tank3
  note: Inputs For Tank1
  CT3 : Inport
  F3 : Inport  Port=2
  E3 : Inport  Port=3
  MR3 : Inport  Port=4
  T3 : Inport  Port=5
  EB3 : Inport  Port=6
  Tank3 : Subsystem
  LL3 : Outport
  wires:
  Tank3/1(LL3) -> LL3/1
  MR3/1 -> Tank3/4(MR3)
  E3/1 -> Tank3/3(E3)
  CT3/1 -> Tank3/1(CT3)
  F3/1 -> Tank3/2(F3)
  EB3/1 -> Tank3/6(EB3)
  T3/1 -> Tank3/5(T3)

== system c00004M_harness/M178 ==
  note: VALUES
      | ---------------------------------
      | ControlType = 1 | 2 | 3
      | FillTank = 0 | 1
      | EmptyTank = 0 | 1
      | ManualReference between 0 and 1
      | Tempreature between 0 and 100
      | EmergencyButton = 0 | 1
      | LiquidLevel between 0 and 1 (hmax)
  note: Inputs For Tank2
  note: NAMES
      | --------------------------------------------
      | CT1 = ControlType Tank 1
      | F1 = Fill Tank 1
      | E1 = Empty Tank 1
      | MR1 = Manual Reference Tank1
      | T1 = Temperature Tank 1
      | EB1 = Emergency Button Tank 1
      | LL1 = Liquid Level 1
  note: Inputs For Tank3
  note: Inputs For Tank1
  CT3 : Inport
  F3 : Inport  Port=2
  E3 : Inport  Port=3
  MR3 : Inport  Port=4
  T3 : Inport  Port=5
  EB3 : Inport  Port=6
  Tank3 : Subsystem
  LL3 : Outport
  wires:
  Tank3/1(LL3) -> LL3/1
  MR3/1 -> Tank3/4(MR3)
  E3/1 -> Tank3/3(E3)
  CT3/1 -> Tank3/1(CT3)
  F3/1 -> Tank3/2(F3)
  EB3/1 -> Tank3/6(EB3)
  T3/1 -> Tank3/5(T3)

== system c00004M_harness/M179 ==
  note: VALUES
      | ---------------------------------
      | ControlType = 1 | 2 | 3
      | FillTank = 0 | 1
      | EmptyTank = 0 | 1
      | ManualReference between 0 and 1
      | Tempreature between 0 and 100
      | EmergencyButton = 0 | 1
      | LiquidLevel between 0 and 1 (hmax)
  note: Inputs For Tank2
  note: NAMES
      | --------------------------------------------
      | CT1 = ControlType Tank 1
      | F1 = Fill Tank 1
      | E1 = Empty Tank 1
      | MR1 = Manual Reference Tank1
      | T1 = Temperature Tank 1
      | EB1 = Emergency Button Tank 1
      | LL1 = Liquid Level 1
  note: Inputs For Tank3
  note: Inputs For Tank1
  CT3 : Inport
  F3 : Inport  Port=2
  E3 : Inport  Port=3
  MR3 : Inport  Port=4
  T3 : Inport  Port=5
  EB3 : Inport  Port=6
  Tank3 : Subsystem
  LL3 : Outport
  wires:
  Tank3/1(LL3) -> LL3/1
  MR3/1 -> Tank3/4(MR3)
  E3/1 -> Tank3/3(E3)
  CT3/1 -> Tank3/1(CT3)
  F3/1 -> Tank3/2(F3)
  EB3/1 -> Tank3/6(EB3)
  T3/1 -> Tank3/5(T3)

== system c00004M_harness/M180 ==
  note: VALUES
      | ---------------------------------
      | ControlType = 1 | 2 | 3
      | FillTank = 0 | 1
      | EmptyTank = 0 | 1
      | ManualReference between 0 and 1
      | Tempreature between 0 and 100
      | EmergencyButton = 0 | 1
      | LiquidLevel between 0 and 1 (hmax)
  note: Inputs For Tank2
  note: NAMES
      | --------------------------------------------
      | CT1 = ControlType Tank 1
      | F1 = Fill Tank 1
      | E1 = Empty Tank 1
      | MR1 = Manual Reference Tank1
      | T1 = Temperature Tank 1
      | EB1 = Emergency Button Tank 1
      | LL1 = Liquid Level 1
  note: Inputs For Tank3
  note: Inputs For Tank1
  CT3 : Inport
  F3 : Inport  Port=2
  E3 : Inport  Port=3
  MR3 : Inport  Port=4
  T3 : Inport  Port=5
  EB3 : Inport  Port=6
  Tank3 : Subsystem
  LL3 : Outport
  wires:
  Tank3/1(LL3) -> LL3/1
  MR3/1 -> Tank3/4(MR3)
  E3/1 -> Tank3/3(E3)
  CT3/1 -> Tank3/1(CT3)
  F3/1 -> Tank3/2(F3)
  EB3/1 -> Tank3/6(EB3)
  T3/1 -> Tank3/5(T3)

== system c00004M_harness/M181 ==
  note: VALUES
      | ---------------------------------
      | ControlType = 1 | 2 | 3
      | FillTank = 0 | 1
      | EmptyTank = 0 | 1
      | ManualReference between 0 and 1
      | Tempreature between 0 and 100
      | EmergencyButton = 0 | 1
      | LiquidLevel between 0 and 1 (hmax)
  note: Inputs For Tank2
  note: NAMES
      | --------------------------------------------
      | CT1 = ControlType Tank 1
      | F1 = Fill Tank 1
      | E1 = Empty Tank 1
      | MR1 = Manual Reference Tank1
      | T1 = Temperature Tank 1
      | EB1 = Emergency Button Tank 1
      | LL1 = Liquid Level 1
  note: Inputs For Tank3
  note: Inputs For Tank1
  CT3 : Inport
  F3 : Inport  Port=2
  E3 : Inport  Port=3
  MR3 : Inport  Port=4
  T3 : Inport  Port=5
  EB3 : Inport  Port=6
  Tank3 : Subsystem
  LL3 : Outport
  wires:
  Tank3/1(LL3) -> LL3/1
  MR3/1 -> Tank3/4(MR3)
  E3/1 -> Tank3/3(E3)
  CT3/1 -> Tank3/1(CT3)
  F3/1 -> Tank3/2(F3)
  EB3/1 -> Tank3/6(EB3)
  T3/1 -> Tank3/5(T3)

== system c00004M_harness/M182 ==
  note: VALUES
      | ---------------------------------
      | ControlType = 1 | 2 | 3
      | FillTank = 0 | 1
      | EmptyTank = 0 | 1
      | ManualReference between 0 and 1
      | Tempreature between 0 and 100
      | EmergencyButton = 0 | 1
      | LiquidLevel between 0 and 1 (hmax)
  note: Inputs For Tank2
  note: NAMES
      | --------------------------------------------
      | CT1 = ControlType Tank 1
      | F1 = Fill Tank 1
      | E1 = Empty Tank 1
      | MR1 = Manual Reference Tank1
      | T1 = Temperature Tank 1
      | EB1 = Emergency Button Tank 1
      | LL1 = Liquid Level 1
  note: Inputs For Tank3
  note: Inputs For Tank1
  CT3 : Inport
  F3 : Inport  Port=2
  E3 : Inport  Port=3
  MR3 : Inport  Port=4
  T3 : Inport  Port=5
  EB3 : Inport  Port=6
  Tank3 : Subsystem
  LL3 : Outport
  wires:
  Tank3/1(LL3) -> LL3/1
  MR3/1 -> Tank3/4(MR3)
  E3/1 -> Tank3/3(E3)
  CT3/1 -> Tank3/1(CT3)
  F3/1 -> Tank3/2(F3)
  EB3/1 -> Tank3/6(EB3)
  T3/1 -> Tank3/5(T3)

== system c00004M_harness/M183 ==
  note: VALUES
      | ---------------------------------
      | ControlType = 1 | 2 | 3
      | FillTank = 0 | 1
      | EmptyTank = 0 | 1
      | ManualReference between 0 and 1
      | Tempreature between 0 and 100
      | EmergencyButton = 0 | 1
      | LiquidLevel between 0 and 1 (hmax)
  note: Inputs For Tank2
  note: NAMES
      | --------------------------------------------
      | CT1 = ControlType Tank 1
      | F1 = Fill Tank 1
      | E1 = Empty Tank 1
      | MR1 = Manual Reference Tank1
      | T1 = Temperature Tank 1
      | EB1 = Emergency Button Tank 1
      | LL1 = Liquid Level 1
  note: Inputs For Tank3
  note: Inputs For Tank1
  CT3 : Inport
  F3 : Inport  Port=2
  E3 : Inport  Port=3
  MR3 : Inport  Port=4
  T3 : Inport  Port=5
  EB3 : Inport  Port=6
  Tank3 : Subsystem
  LL3 : Outport
  wires:
  Tank3/1(LL3) -> LL3/1
  MR3/1 -> Tank3/4(MR3)
  E3/1 -> Tank3/3(E3)
  CT3/1 -> Tank3/1(CT3)
  F3/1 -> Tank3/2(F3)
  EB3/1 -> Tank3/6(EB3)
  T3/1 -> Tank3/5(T3)

== system c00004M_harness/M184 ==
  note: VALUES
      | ---------------------------------
      | ControlType = 1 | 2 | 3
      | FillTank = 0 | 1
      | EmptyTank = 0 | 1
      | ManualReference between 0 and 1
      | Tempreature between 0 and 100
      | EmergencyButton = 0 | 1
      | LiquidLevel between 0 and 1 (hmax)
  note: Inputs For Tank2
  note: NAMES
      | --------------------------------------------
      | CT1 = ControlType Tank 1
      | F1 = Fill Tank 1
      | E1 = Empty Tank 1
      | MR1 = Manual Reference Tank1
      | T1 = Temperature Tank 1
      | EB1 = Emergency Button Tank 1
      | LL1 = Liquid Level 1
  note: Inputs For Tank3
  note: Inputs For Tank1
  CT3 : Inport
  F3 : Inport  Port=2
  E3 : Inport  Port=3
  MR3 : Inport  Port=4
  T3 : Inport  Port=5
  EB3 : Inport  Port=6
  Tank3 : Subsystem
  LL3 : Outport
  wires:
  Tank3/1(LL3) -> LL3/1
  MR3/1 -> Tank3/4(MR3)
  E3/1 -> Tank3/3(E3)
  CT3/1 -> Tank3/1(CT3)
  F3/1 -> Tank3/2(F3)
  EB3/1 -> Tank3/6(EB3)
  T3/1 -> Tank3/5(T3)

== system c00004M_harness/M185 ==
  note: VALUES
      | ---------------------------------
      | ControlType = 1 | 2 | 3
      | FillTank = 0 | 1
      | EmptyTank = 0 | 1
      | ManualReference between 0 and 1
      | Tempreature between 0 and 100
      | EmergencyButton = 0 | 1
      | LiquidLevel between 0 and 1 (hmax)
  note: Inputs For Tank2
  note: NAMES
      | --------------------------------------------
      | CT1 = ControlType Tank 1
      | F1 = Fill Tank 1
      | E1 = Empty Tank 1
      | MR1 = Manual Reference Tank1
      | T1 = Temperature Tank 1
      | EB1 = Emergency Button Tank 1
      | LL1 = Liquid Level 1
  note: Inputs For Tank3
  note: Inputs For Tank1
  CT3 : Inport
  F3 : Inport  Port=2
  E3 : Inport  Port=3
  MR3 : Inport  Port=4
  T3 : Inport  Port=5
  EB3 : Inport  Port=6
  Tank3 : Subsystem
  LL3 : Outport
  wires:
  Tank3/1(LL3) -> LL3/1
  MR3/1 -> Tank3/4(MR3)
  E3/1 -> Tank3/3(E3)
  CT3/1 -> Tank3/1(CT3)
  F3/1 -> Tank3/2(F3)
  EB3/1 -> Tank3/6(EB3)
  T3/1 -> Tank3/5(T3)

== system c00004M_harness/M186 ==
  note: VALUES
      | ---------------------------------
      | ControlType = 1 | 2 | 3
      | FillTank = 0 | 1
      | EmptyTank = 0 | 1
      | ManualReference between 0 and 1
      | Tempreature between 0 and 100
      | EmergencyButton = 0 | 1
      | LiquidLevel between 0 and 1 (hmax)
  note: Inputs For Tank2
  note: NAMES
      | --------------------------------------------
      | CT1 = ControlType Tank 1
      | F1 = Fill Tank 1
      | E1 = Empty Tank 1
      | MR1 = Manual Reference Tank1
      | T1 = Temperature Tank 1
      | EB1 = Emergency Button Tank 1
      | LL1 = Liquid Level 1
  note: Inputs For Tank3
  note: Inputs For Tank1
  CT3 : Inport
  F3 : Inport  Port=2
  E3 : Inport  Port=3
  MR3 : Inport  Port=4
  T3 : Inport  Port=5
  EB3 : Inport  Port=6
  Tank3 : Subsystem
  LL3 : Outport
  wires:
  Tank3/1(LL3) -> LL3/1
  MR3/1 -> Tank3/4(MR3)
  E3/1 -> Tank3/3(E3)
  CT3/1 -> Tank3/1(CT3)
  F3/1 -> Tank3/2(F3)
  EB3/1 -> Tank3/6(EB3)
  T3/1 -> Tank3/5(T3)

== system c00004M_harness/M187 ==
  note: VALUES
      | ---------------------------------
      | ControlType = 1 | 2 | 3
      | FillTank = 0 | 1
      | EmptyTank = 0 | 1
      | ManualReference between 0 and 1
      | Tempreature between 0 and 100
      | EmergencyButton = 0 | 1
      | LiquidLevel between 0 and 1 (hmax)
  note: Inputs For Tank2
  note: NAMES
      | --------------------------------------------
      | CT1 = ControlType Tank 1
      | F1 = Fill Tank 1
      | E1 = Empty Tank 1
      | MR1 = Manual Reference Tank1
      | T1 = Temperature Tank 1
      | EB1 = Emergency Button Tank 1
      | LL1 = Liquid Level 1
  note: Inputs For Tank3
  note: Inputs For Tank1
  CT3 : Inport
  F3 : Inport  Port=2
  E3 : Inport  Port=3
  MR3 : Inport  Port=4
  T3 : Inport  Port=5
  EB3 : Inport  Port=6
  Tank3 : Subsystem
  LL3 : Outport
  wires:
  Tank3/1(LL3) -> LL3/1
  MR3/1 -> Tank3/4(MR3)
  E3/1 -> Tank3/3(E3)
  CT3/1 -> Tank3/1(CT3)
  F3/1 -> Tank3/2(F3)
  EB3/1 -> Tank3/6(EB3)
  T3/1 -> Tank3/5(T3)

== system c00004M_harness/M188 ==
  note: VALUES
      | ---------------------------------
      | ControlType = 1 | 2 | 3
      | FillTank = 0 | 1
      | EmptyTank = 0 | 1
      | ManualReference between 0 and 1
      | Tempreature between 0 and 100
      | EmergencyButton = 0 | 1
      | LiquidLevel between 0 and 1 (hmax)
  note: Inputs For Tank2
  note: NAMES
      | --------------------------------------------
      | CT1 = ControlType Tank 1
      | F1 = Fill Tank 1
      | E1 = Empty Tank 1
      | MR1 = Manual Reference Tank1
      | T1 = Temperature Tank 1
      | EB1 = Emergency Button Tank 1
      | LL1 = Liquid Level 1
  note: Inputs For Tank3
  note: Inputs For Tank1
  CT3 : Inport
  F3 : Inport  Port=2
  E3 : Inport  Port=3
  MR3 : Inport  Port=4
  T3 : Inport  Port=5
  EB3 : Inport  Port=6
  Tank3 : Subsystem
  LL3 : Outport
  wires:
  Tank3/1(LL3) -> LL3/1
  MR3/1 -> Tank3/4(MR3)
  E3/1 -> Tank3/3(E3)
  CT3/1 -> Tank3/1(CT3)
  F3/1 -> Tank3/2(F3)
  EB3/1 -> Tank3/6(EB3)
  T3/1 -> Tank3/5(T3)

== system c00004M_harness/M189 ==
  note: VALUES
      | ---------------------------------
      | ControlType = 1 | 2 | 3
      | FillTank = 0 | 1
      | EmptyTank = 0 | 1
      | ManualReference between 0 and 1
      | Tempreature between 0 and 100
      | EmergencyButton = 0 | 1
      | LiquidLevel between 0 and 1 (hmax)
  note: Inputs For Tank2
  note: NAMES
      | --------------------------------------------
      | CT1 = ControlType Tank 1
      | F1 = Fill Tank 1
      | E1 = Empty Tank 1
      | MR1 = Manual Reference Tank1
      | T1 = Temperature Tank 1
      | EB1 = Emergency Button Tank 1
      | LL1 = Liquid Level 1
  note: Inputs For Tank3
  note: Inputs For Tank1
  CT3 : Inport
  F3 : Inport  Port=2
  E3 : Inport  Port=3
  MR3 : Inport  Port=4
  T3 : Inport  Port=5
  EB3 : Inport  Port=6
  Tank3 : Subsystem
  LL3 : Outport
  wires:
  Tank3/1(LL3) -> LL3/1
  MR3/1 -> Tank3/4(MR3)
  E3/1 -> Tank3/3(E3)
  CT3/1 -> Tank3/1(CT3)
  F3/1 -> Tank3/2(F3)
  EB3/1 -> Tank3/6(EB3)
  T3/1 -> Tank3/5(T3)

== system c00004M_harness/M190 ==
  note: VALUES
      | ---------------------------------
      | ControlType = 1 | 2 | 3
      | FillTank = 0 | 1
      | EmptyTank = 0 | 1
      | ManualReference between 0 and 1
      | Tempreature between 0 and 100
      | EmergencyButton = 0 | 1
      | LiquidLevel between 0 and 1 (hmax)
  note: Inputs For Tank2
  note: NAMES
      | --------------------------------------------
      | CT1 = ControlType Tank 1
      | F1 = Fill Tank 1
      | E1 = Empty Tank 1
      | MR1 = Manual Reference Tank1
      | T1 = Temperature Tank 1
      | EB1 = Emergency Button Tank 1
      | LL1 = Liquid Level 1
  note: Inputs For Tank3
  note: Inputs For Tank1
  CT3 : Inport
  F3 : Inport  Port=2
  E3 : Inport  Port=3
  MR3 : Inport  Port=4
  T3 : Inport  Port=5
  EB3 : Inport  Port=6
  Tank3 : Subsystem
  LL3 : Outport
  wires:
  Tank3/1(LL3) -> LL3/1
  MR3/1 -> Tank3/4(MR3)
  E3/1 -> Tank3/3(E3)
  CT3/1 -> Tank3/1(CT3)
  F3/1 -> Tank3/2(F3)
  EB3/1 -> Tank3/6(EB3)
  T3/1 -> Tank3/5(T3)

== system c00004M_harness/M191 ==
  note: VALUES
      | ---------------------------------
      | ControlType = 1 | 2 | 3
      | FillTank = 0 | 1
      | EmptyTank = 0 | 1
      | ManualReference between 0 and 1
      | Tempreature between 0 and 100
      | EmergencyButton = 0 | 1
      | LiquidLevel between 0 and 1 (hmax)
  note: Inputs For Tank2
  note: NAMES
      | --------------------------------------------
      | CT1 = ControlType Tank 1
      | F1 = Fill Tank 1
      | E1 = Empty Tank 1
      | MR1 = Manual Reference Tank1
      | T1 = Temperature Tank 1
      | EB1 = Emergency Button Tank 1
      | LL1 = Liquid Level 1
  note: Inputs For Tank3
  note: Inputs For Tank1
  CT3 : Inport
  F3 : Inport  Port=2
  E3 : Inport  Port=3
  MR3 : Inport  Port=4
  T3 : Inport  Port=5
  EB3 : Inport  Port=6
  Tank3 : Subsystem
  LL3 : Outport
  wires:
  Tank3/1(LL3) -> LL3/1
  MR3/1 -> Tank3/4(MR3)
  E3/1 -> Tank3/3(E3)
  CT3/1 -> Tank3/1(CT3)
  F3/1 -> Tank3/2(F3)
  EB3/1 -> Tank3/6(EB3)
  T3/1 -> Tank3/5(T3)

== system c00004M_harness/M192 ==
  note: VALUES
      | ---------------------------------
      | ControlType = 1 | 2 | 3
      | FillTank = 0 | 1
      | EmptyTank = 0 | 1
      | ManualReference between 0 and 1
      | Tempreature between 0 and 100
      | EmergencyButton = 0 | 1
      | LiquidLevel between 0 and 1 (hmax)
  note: Inputs For Tank2
  note: NAMES
      | --------------------------------------------
      | CT1 = ControlType Tank 1
      | F1 = Fill Tank 1
      | E1 = Empty Tank 1
      | MR1 = Manual Reference Tank1
      | T1 = Temperature Tank 1
      | EB1 = Emergency Button Tank 1
      | LL1 = Liquid Level 1
  note: Inputs For Tank3
  note: Inputs For Tank1
  CT3 : Inport
  F3 : Inport  Port=2
  E3 : Inport  Port=3
  MR3 : Inport  Port=4
  T3 : Inport  Port=5
  EB3 : Inport  Port=6
  Tank3 : Subsystem
  LL3 : Outport
  wires:
  Tank3/1(LL3) -> LL3/1
  MR3/1 -> Tank3/4(MR3)
  E3/1 -> Tank3/3(E3)
  CT3/1 -> Tank3/1(CT3)
  F3/1 -> Tank3/2(F3)
  EB3/1 -> Tank3/6(EB3)
  T3/1 -> Tank3/5(T3)

== system c00004M_harness/M193 ==
  note: VALUES
      | ---------------------------------
      | ControlType = 1 | 2 | 3
      | FillTank = 0 | 1
      | EmptyTank = 0 | 1
      | ManualReference between 0 and 1
      | Tempreature between 0 and 100
      | EmergencyButton = 0 | 1
      | LiquidLevel between 0 and 1 (hmax)
  note: Inputs For Tank2
  note: NAMES
      | --------------------------------------------
      | CT1 = ControlType Tank 1
      | F1 = Fill Tank 1
      | E1 = Empty Tank 1
      | MR1 = Manual Reference Tank1
      | T1 = Temperature Tank 1
      | EB1 = Emergency Button Tank 1
      | LL1 = Liquid Level 1
  note: Inputs For Tank3
  note: Inputs For Tank1
  CT3 : Inport
  F3 : Inport  Port=2
  E3 : Inport  Port=3
  MR3 : Inport  Port=4
  T3 : Inport  Port=5
  EB3 : Inport  Port=6
  Tank3 : Subsystem
  LL3 : Outport
  wires:
  Tank3/1(LL3) -> LL3/1
  MR3/1 -> Tank3/4(MR3)
  E3/1 -> Tank3/3(E3)
  CT3/1 -> Tank3/1(CT3)
  F3/1 -> Tank3/2(F3)
  EB3/1 -> Tank3/6(EB3)
  T3/1 -> Tank3/5(T3)
